simulink model "ap_12B"  (Simulink 8.0)
settings: Solver=ode3  StartTime=0.0  StopTime=100  FixedStep=Ts  RelTol=1e-3
undefined symbols (not defined in the file): beaver_b, beaver_c, beaver_mass, beaver_S, Cl0, Cl_alpha2_dpt, Cl_beta, Cl_da, Cl_da_alpha, Cl_dr, Cl_p, Cl_r, Cm0, Cm_alpha, Cm_alpha2, Cm_beta2, Cm_de, Cm_df, Cm_dpt, Cm_q, Cm_r, Cn0, Cn_beta, Cn_beta3, Cn_da, Cn_dpt3, Cn_dr, Cn_p, Cn_q, Cn_r, Cx0, Cx_alpha, Cx_alpha2, Cx_alpha3, Cx_df, Cx_df_alpha, Cx_dpt, Cx_dpt2_alpha, Cx_dr, Cx_q, Cy0, Cy_beta, Cy_da, Cy_dr, Cy_dr_alpha, Cy_p, Cy_r, Cz0, Cz_alpha, Cz_alpha3, Cz_de, Cz_de_beta, Cz_df, Cz_df_alpha, Cz_dpt, Cz_q, d2r, fin_act_1, fin_act_2, fin_act_3 ... (+23)
libraries: simulink x12, aerolibtransform2 x9, aerolibutil x7, aerolibasang x7, aerolibadynsys x3, aerolib6dofsys x2, aerolib6dof2 x1
(part 2 of 3)

== system ap_12B/DeHavilland Beaver Airframe/Aircraft Dynamics/Total Forces  and Moments ==
  EnvirBus : Inport
  Pilot : Inport  Port=2
  DCM : Inport  Port=3
  FltParams : Inport  Port=4
  Actuators : Subsystem
  Aerodynamics : Subsystem
  Bus Selector4 : BusSelector  OutputSignals=rho,g
  "Engine " : Subsystem
  Forces and Moments : Subsystem
  "Gravity " : Subsystem
  "Pilot " : InportShadow  Port=2
  Sum : Sum  Inputs=|++  SaturateOnIntegerOverflow=on  InputSameDT=on  OutDataTypeStr=Inherit: Same as first input
  Total Force : Outport
  Total Moment : Outport  Port=2
  wires:
  Forces and Moments/1(XYZ) -> Sum/1
  "Engine "/1(Engine Coefficients) -> Forces and Moments/3(Engine Coefficients)
  "Gravity "/1(Fgrav) -> Sum/2
  Aerodynamics/1(Aero Coefficients) -> Forces and Moments/1(Aero Coefficients)
  Pilot/1 -> Actuators/1(Pilot)
  Bus Selector4/1 -> "Engine "/3(rho)  "<rho>"
  DCM/1 -> "Gravity "/2(DCM)
  Bus Selector4/2 -> "Gravity "/1(g)  "<g>"
  Sum/1 -> Total Force/1  "Ftot"
  Forces and Moments/2(LMN) -> Total Moment/1  "Mtot"
  "Pilot "/1 -> "Engine "/2(Pilot)
  FltParams/1 -> Forces and Moments/2(Fltparams), "Engine "/1(Fltparams), Aerodynamics/2(FltParams)
  Actuators/1(uaero-out) -> Aerodynamics/1(Uaero)
  EnvirBus/1 -> Bus Selector4/1

== system ap_12B/DeHavilland Beaver Airframe/Calculate Parameters/ Incidence, Sideslip,  & Airspeed ==
  Vb : Inport
  Airspeed : Sqrt  AlgorithmType=Newton-Raphson  SaturateOnIntegerOverflow=on
  Incidence : Trigonometry  Operator=atan2
  Product : Product  Inputs=*/  SaturateOnIntegerOverflow=on  OutDataTypeStr=Inherit: Same as first input
  Sideslip : Trigonometry  Operator=asin
  Subsystem : aerolibasang/Incidence, Sideslip, & Airspeed/Subsystem
  Subsystem1 : aerolibasang/Incidence, Sideslip, & Airspeed/Subsystem1
  dot : aerolibasang/Incidence, Sideslip, & Airspeed/dot
  Alpha : Outport  InitialOutput=0
  Beta : Outport  Port=2  InitialOutput=0
  V : Outport  Port=3  InitialOutput=0
  wires:
  Sideslip/1 -> Beta/1
  Subsystem1/1 -> Product/1
  Product/1 -> Sideslip/1
  Subsystem/1 -> Incidence/1
  Subsystem/2 -> Incidence/2
  dot/1 -> Airspeed/1
  Airspeed/1 -> V/1, Product/2
  Incidence/1 -> Alpha/1
  Vb/1 -> Subsystem/1, dot/1, Subsystem1/1

== system ap_12B/DeHavilland Beaver Airframe/Calculate Parameters/Dynamic Pressure ==
  Velocity : Inport
  Air Density : Inport  Port=2
  1/2rhoV^2 : Gain  Gain=0.5  SaturateOnIntegerOverflow=on  OutDataTypeStr=Inherit: Same as input  ParamDataTypeStr=Inherit: Same as input
  Product2 : Product  SaturateOnIntegerOverflow=on  InputSameDT=on  OutDataTypeStr=Inherit: Same as first input
  dot : aerolibasang/Dynamic Pressure/dot
  qbar : Outport  InitialOutput=0
  wires:
  1/2rhoV^2/1 -> qbar/1
  Air Density/1 -> Product2/2
  dot/1 -> Product2/1
  Product2/1 -> 1/2rhoV^2/1
  Velocity/1 -> dot/1

== system ap_12B/Sensors/Air Data Sensor/ Incidence, Sideslip,  & Airspeed ==
  Vb : Inport
  Airspeed : Sqrt  AlgorithmType=Newton-Raphson  SaturateOnIntegerOverflow=on
  Gain : Gain  Gain=180/pi
  Gain1 : Gain  Gain=180/pi
  Incidence : Trigonometry  Operator=atan2
  Product : Product  Inputs=*/  SaturateOnIntegerOverflow=on  OutDataTypeStr=Inherit: Same as first input
  Scope : Scope
      settings: SaveName=ScopeData24
  Scope1 : Scope
      settings: SaveName=ScopeData25
  Sideslip : Trigonometry  Operator=asin
  Subsystem : aerolibasang/Incidence, Sideslip, & Airspeed/Subsystem
  Subsystem1 : aerolibasang/Incidence, Sideslip, & Airspeed/Subsystem1
  dot : aerolibasang/Incidence, Sideslip, & Airspeed/dot
  Alpha : Outport  InitialOutput=0
  Beta : Outport  Port=2  InitialOutput=0
  V : Outport  Port=3  InitialOutput=0
  wires:
  Sideslip/1 -> Gain1/1, Beta/1
  Subsystem1/1 -> Product/1
  Product/1 -> Sideslip/1
  Subsystem/1 -> Incidence/1
  Subsystem/2 -> Incidence/2
  dot/1 -> Airspeed/1
  Airspeed/1 -> V/1, Product/2
  Incidence/1 -> Gain/1, Alpha/1
  Vb/1 -> Subsystem/1, dot/1, Subsystem1/1
  Gain/1 -> Scope/1
  Gain1/1 -> Scope1/1

== system ap_12B/Sensors/Air Data Sensor/ic1 ==
  u : Inport
  ic : Inport  Port=2
  Constant : Constant
  Switch : Switch  Criteria=u2 ~= 0
  Unit Delay : UnitDelay  SampleTime=-1
  y : Outport
  wires:
  Switch/1 -> y/1
  u/1 -> Switch/1
  ic/1 -> Switch/3
  Constant/1 -> Unit Delay/1
  Unit Delay/1 -> Switch/2

== system ap_12B/Sensors/Air Data Sensor/ic2 ==
  u : Inport
  ic : Inport  Port=2
  Constant : Constant
  Switch : Switch  Criteria=u2 ~= 0
  Unit Delay : UnitDelay  SampleTime=-1
  y : Outport
  wires:
  ic/1 -> Switch/3
  u/1 -> Switch/1
  Switch/1 -> y/1
  Constant/1 -> Unit Delay/1
  Unit Delay/1 -> Switch/2

== system ap_12B/Sensors/Air Data Sensor/ic3 ==
  u : Inport
  ic : Inport  Port=2
  Constant1 : Constant
  Switch : Switch  Criteria=u2 ~= 0
  Unit Delay1 : UnitDelay  SampleTime=-1
  y : Outport
  wires:
  ic/1 -> Switch/3
  u/1 -> Switch/1
  Switch/1 -> y/1
  Constant1/1 -> Unit Delay1/1
  Unit Delay1/1 -> Switch/2

== system ap_12B/Sensors/Inertial Data Sensor/ic ==
  u : Inport
  ic : Inport  Port=2
  Constant : Constant
  Switch : Switch  Criteria=u2 ~= 0
  Unit Delay : UnitDelay  SampleTime=-1
  y : Outport
  wires:
  Switch/1 -> y/1
  u/1 -> Switch/1
  ic/1 -> Switch/3
  Constant/1 -> Unit Delay/1
  Unit Delay/1 -> Switch/2

== system ap_12B/Sensors/Inertial Data Sensor/ic1 ==
  u : Inport
  ic : Inport  Port=2
  Constant : Constant
  Switch : Switch  Criteria=u2 ~= 0
  Unit Delay : UnitDelay  SampleTime=-1
  y : Outport
  wires:
  ic/1 -> Switch/3
  u/1 -> Switch/1
  Switch/1 -> y/1
  Constant/1 -> Unit Delay/1
  Unit Delay/1 -> Switch/2

== system ap_12B/Sensors/Inertial Data Sensor/ic2 ==
  u : Inport
  ic : Inport  Port=2
  Constant : Constant
  Switch : Switch  Criteria=u2 ~= 0
  Unit Delay : UnitDelay  SampleTime=-1
  y : Outport
  wires:
  Switch/1 -> y/1
  u/1 -> Switch/1
  ic/1 -> Switch/3
  Constant/1 -> Unit Delay/1
  Unit Delay/1 -> Switch/2

== system ap_12B/Sensors/Inertial Data Sensor/ic3 ==
  u : Inport
  ic : Inport  Port=2
  Constant : Constant
  Switch : Switch  Criteria=u2 ~= 0
  Unit Delay : UnitDelay  SampleTime=-1
  y : Outport
  wires:
  ic/1 -> Switch/3
  u/1 -> Switch/1
  Switch/1 -> y/1
  Constant/1 -> Unit Delay/1
  Unit Delay/1 -> Switch/2

== system ap_12B/Autopilot/Pitch_Autopilot/Altitude Mode/Rate Limiter ==
  note: Y(k)
  note: U(k)
  up : Inport
  u : Inport  Port=2
  lo : Inport  Port=3
  Constant1 : Constant  Value=Ts
  Delay Input2 : UnitDelay  Description=Store in Global RAM  DisableCoverage=on  SampleTime=-1
  Difference Inputs1 : Sum  Description=Add in CPU  DisableCoverage=on  Inputs=+-  OutDataTypeStr=Inherit: Inherit via back propagation
  Difference Inputs2 : Sum  Description=Add in CPU  OutDataTypeStr=Inherit: Inherit via back propagation
  Saturation Dynamic : simulink/Discontinuities/Saturation Dynamic  OutMin=[]  OutMax=[]  OutDataTypeStr=Inherit: Same as second input  OutDataType=fixdt(1, 16)  OutScaling=2^-10  DoSatur=off
  delta fall limit : Product  DisableCoverage=on  Inputs=**  OutDataTypeStr=Inherit: Inherit via back propagation  SaturateOnIntegerOverflow=on
  delta rise limit : Product  DisableCoverage=on  Inputs=**  OutDataTypeStr=Inherit: Inherit via back propagation  SaturateOnIntegerOverflow=on
  Y : Outport  InitialOutput=0
  wires:
  Difference Inputs1/1 -> Saturation Dynamic/2  "( U(k) - Y(k-1) )"
  u/1 -> Difference Inputs1/1
  delta fall limit/1 -> Saturation Dynamic/3
  Saturation Dynamic/1 -> Difference Inputs2/1
  Delay Input2/1 -> Difference Inputs1/2, Difference Inputs2/2  "Y(k-1)"
  Difference Inputs2/1 -> Y/1, Delay Input2/1
  up/1 -> delta rise limit/1
  delta rise limit/1 -> Saturation Dynamic/1
  lo/1 -> delta fall limit/1
  Constant1/1 -> delta rise limit/2, delta fall limit/2

== system ap_12B/Autopilot/Pitch_Autopilot/Altitude Mode/ResetIntegratorInternal ==
  note: ic
  note: Level Reset Integration With Saturation
      | y(n) = y(n-1) + K*Ts*u(n-1)
  U : Inport
  R : Inport  Port=2
  IC : Inport  Port=3
  Constant : Constant  Value=0.2
  Constant1 : Constant  Value=Ts
  Product : Product  RndMeth=Zero
  Product1 : Product  RndMeth=Zero
  Saturation : Saturate  UpperLimit=20  LowerLimit=-20
  Sum3 : Sum
  Switch : Switch  Criteria=u2 ~= 0
  Switch1 : Switch  Criteria=u2 ~= 0
  X : UnitDelay  SampleTime=Ts
  Y : Outport
  wires:
  Product1/1 -> Sum3/1
  U/1 -> Product1/2
  Sum3/1 -> Switch1/3
  Product/1 -> Product1/1
  Switch/1 -> Saturation/1
  IC/1 -> Switch1/1, Switch/1
  Constant1/1 -> Product/2  "deltaT"
  Switch1/1 -> X/1
  Constant/1 -> Product/1  "gain"
  Saturation/1 -> Y/1, Sum3/2
  R/1 -> Switch1/2, Switch/2
  X/1 -> Switch/3

== system ap_12B/Autopilot/Pitch_Autopilot/Basic Pitch Mode/ResetIntegratorInternal ==
  note: ic
  note: Level Reset Integration With Saturation
      | y(n) = y(n-1) + K*Ts*u(n-1)
  U : Inport
  R : Inport  Port=2
  Constant : Constant  Value=1.0
  Constant1 : Constant  Value=Ts
  Constant2 : Constant  Value=0.0
  Product : Product  RndMeth=Zero
  Product1 : Product  RndMeth=Zero
  Saturation : Saturate  UpperLimit=5  LowerLimit=-5
  Sum3 : Sum
  Switch : Switch  Criteria=u2 ~= 0
  Switch1 : Switch  Criteria=u2 ~= 0
  X : UnitDelay  SampleTime=Ts
  Y : Outport
  wires:
  Product1/1 -> Sum3/1
  U/1 -> Product1/2
  Sum3/1 -> Switch1/3
  Product/1 -> Product1/1
  Switch/1 -> Saturation/1
  Constant2/1 -> Switch1/1, Switch/1
  Constant1/1 -> Product/2  "deltaT"
  Switch1/1 -> X/1
  Constant/1 -> Product/1  "gain"
  Saturation/1 -> Y/1, Sum3/2
  R/1 -> Switch1/2, Switch/2
  X/1 -> Switch/3

== system ap_12B/Autopilot/Pitch_Autopilot/Pitch Reference/latch ==
  note: Xold
  note: Enable
  u : Inport
  E : Inport  Port=2
  Enable : Switch  Criteria=u2 ~= 0  OutDataTypeStr=Inherit: Inherit via back propagation  ZeroCross=off
  FixPt Unit Delay1 : UnitDelay  SampleTime=Ts  HasFrameUpgradeWarning=off
  y : Outport
  wires:
  FixPt Unit Delay1/1 -> y/1, Enable/3
  Enable/1 -> FixPt Unit Delay1/1  "Xnew"
  E/1 -> Enable/2
  u/1 -> Enable/1

== system ap_12B/Autopilot/Roll_Autopilot/Basic Roll Mode/ResetIntegratorInternal ==
  note: ic
  note: Level Reset Integration With Saturation
      | y(n) = y(n-1) + K*Ts*u(n-1)
  U : Inport
  R : Inport  Port=2
  Constant : Constant  Value=1.0
  Constant1 : Constant  Value=Ts
  Constant2 : Constant  Value=0.0
  Product : Product  RndMeth=Zero
  Product1 : Product  RndMeth=Zero
  Saturation : Saturate  UpperLimit=5  LowerLimit=-5
  Sum3 : Sum
  Switch : Switch  Criteria=u2 ~= 0
  Switch1 : Switch  Criteria=u2 ~= 0
  X : UnitDelay  SampleTime=Ts
  Y : Outport
  wires:
  Product1/1 -> Sum3/1
  U/1 -> Product1/2
  Sum3/1 -> Switch1/3
  Product/1 -> Product1/1
  Switch/1 -> Saturation/1
  Constant2/1 -> Switch1/1, Switch/1
  Constant1/1 -> Product/2  "deltaT"
  Switch1/1 -> X/1
  Constant/1 -> Product/1  "gain"
  Saturation/1 -> Y/1, Sum3/2
  R/1 -> Switch1/2, Switch/2
  X/1 -> Switch/3

== system ap_12B/Autopilot/Roll_Autopilot/Heading Mode/angle diff ==
  plus : Inport  OutDataTypeStr=double
  minus : Inport  Port=2  OutDataTypeStr=double
  abs : Abs  ZeroCross=off
  constant : Constant  Value=180
  constant1 : Constant  Value=360
  floor : Rounding
  product : Product  RndMeth=Zero  InputSameDT=on  OutDataTypeStr=Inherit: Same as first input
  product1 : Product  Inputs=*/  RndMeth=Zero  InputSameDT=on  OutDataTypeStr=Inherit: Same as first input
  product2 : Product  RndMeth=Zero  InputSameDT=on  OutDataTypeStr=Inherit: Same as first input
  signum : Signum  ZeroCross=off
  sum : Sum  Inputs=|+-  RndMeth=Zero  InputSameDT=on  OutDataTypeStr=Inherit: Same as first input
  sum1 : Sum  Inputs=|+-  RndMeth=Zero  InputSameDT=on  OutDataTypeStr=Inherit: Same as first input
  sum2 : Sum  Inputs=|++  RndMeth=Zero  InputSameDT=on  OutDataTypeStr=Inherit: Same as first input
  diff : Outport
  wires:
  product2/1 -> product/2
  product/1 -> sum1/2
  sum2/1 -> product1/1
  constant/1 -> sum2/2
  sum1/1 -> diff/1
  signum/1 -> product/1
  floor/1 -> product2/1
  minus/1 -> sum/2
  plus/1 -> sum/1
  product1/1 -> floor/1
  sum/1 -> sum1/1, abs/1, signum/1
  abs/1 -> sum2/1
  constant1/1 -> product2/2, product1/2

== system ap_12B/Autopilot/Roll_Autopilot/Roll Reference/latch ==
  note: Xold
  note: Enable
  u : Inport
  E : Inport  Port=2
  Enable : Switch  Criteria=u2 ~= 0  OutDataTypeStr=Inherit: Inherit via back propagation  ZeroCross=off
  FixPt Unit Delay1 : UnitDelay  SampleTime=Ts  HasFrameUpgradeWarning=off
  y : Outport
  wires:
  FixPt Unit Delay1/1 -> y/1, Enable/3
  Enable/1 -> FixPt Unit Delay1/1  "Xnew"
  E/1 -> Enable/2
  u/1 -> Enable/1

== system ap_12B/DeHavilland Beaver Airframe/Aircraft Dynamics/6DoF (Quaternion)/3x3 CrossProduct ==
  A : Inport
  B : Inport  Port=2
  A_1 : InportShadow
  B_1 : InportShadow  Port=2
  Subsystem : aerolibutil/3x3 Cross Product/Subsystem
  Subsystem1 : aerolibutil/3x3 Cross Product/Subsystem1
  Sum : Sum  Inputs=+|-  SaturateOnIntegerOverflow=on  InputSameDT=on  OutDataTypeStr=Inherit: Same as first input
  C : Outport
  wires:
  Subsystem/1 -> Sum/1
  Subsystem1/1 -> Sum/2
  B/1 -> Subsystem/2
  A/1 -> Subsystem/1
  B_1/1 -> Subsystem1/2
  A_1/1 -> Subsystem1/1
  Sum/1 -> C/1

== system ap_12B/DeHavilland Beaver Airframe/Aircraft Dynamics/6DoF (Quaternion)/Calculate DCM & Euler Angles ==
  p q r : Inport
  Initial Euler Angles : Constant  Value="[0    0.1303    1.9722]"
  Quaternions to  Direction Cosine Matrix : Subsystem
  Quaternions to Rotation Angles (ZYX) : Subsystem
  ResetIntegratorInternal1 : Subsystem
  Rotation Angles to Quats (ZYX) : Subsystem
  Selector : Selector  InputPortWidth=3  IndexOptions=Index vector (dialog)  Indices=[3 2 1]  OutputSizes=1
  Selector1 : Selector  InputPortWidth=3  IndexOptions=Index vector (dialog)  Indices=[3 2 1]  OutputSizes=1
  ic3 : Subsystem
  qd : Subsystem
  DCM : Outport
  Euler : Outport  Port=2
  wires:
  Selector1/1 -> Rotation Angles to Quats (ZYX)/1("R1, R2, R3")
  Selector/1 -> Euler/1
  Quaternions to Rotation Angles (ZYX)/1(R1,R2,R3) -> Selector/1
  Quaternions to  Direction Cosine Matrix/1(DCM) -> DCM/1
  p q r/1 -> qd/1(p q r)
  Initial Euler Angles/1 -> Selector1/1
  ResetIntegratorInternal1/1(Y) -> Quaternions to  Direction Cosine Matrix/1(Quat), qd/2(q0 q1 q2 q3), Quaternions to Rotation Angles (ZYX)/1(q)
  qd/1(qdot) -> ResetIntegratorInternal1/1(U)
  ic3/1(R) -> ResetIntegratorInternal1/2(R)
  ic3/2(IC) -> ResetIntegratorInternal1/3(IC)
  Rotation Angles to Quats (ZYX)/1(Quat) -> ic3/1(ic)

== system ap_12B/DeHavilland Beaver Airframe/Aircraft Dynamics/6DoF (Quaternion)/Calculate omega_dot ==
  p q r : Inport
  "I, I_dot" : Inport  Port=2
  Moments : Inport  Port=3
  3x3 CrossProduct : Subsystem
  I x w : aerolib6dofsys/Calculate omega_dot/I x w
  I x w1 : aerolib6dofsys/Calculate omega_dot/I x w1
  Product2 : Product  Inputs=*/  Multiplication=Matrix(*)  SaturateOnIntegerOverflow=on  OutDataTypeStr=Inherit: Same as first input
  Reshape : Reshape
  Reshape1 : Reshape  OutputDimensionality=Row vector (2-D)
  Selector : Selector  NumberOfDimensions=2  InputPortWidth=2  IndexOptions=Index vector (dialog),Select all  Indices=1:3,-1  OutputSizes=1
  Selector1 : Selector  NumberOfDimensions=2  InputPortWidth=2  IndexOptions=Index vector (dialog),Select all  Indices=4:6,-1  OutputSizes=1
  Selector2 : Selector  NumberOfDimensions=2  InputPortWidth=2  IndexOptions=Index vector (dialog),Select all  Indices=1:3,-1  OutputSizes=1
  Sum2 : Sum  Inputs=+--  SaturateOnIntegerOverflow=on
  pdot qdot rdot : Outport
  wires:
  Reshape1/1 -> Product2/1
  I x w/1 -> 3x3 CrossProduct/2(B)
  3x3 CrossProduct/1(C) -> Sum2/3
  Selector1/1 -> I x w1/1
  I x w1/1 -> Sum2/2
  Moments/1 -> Sum2/1
  Sum2/1 -> Reshape1/1
  Product2/1 -> Reshape/1
  p q r/1 -> 3x3 CrossProduct/1(A), I x w1/2, I x w/1
  "I, I_dot"/1 -> Selector2/1, Selector/1, Selector1/1
  Selector2/1 -> Product2/2
  Selector/1 -> I x w/2
  Reshape/1 -> pdot qdot rdot/1

== system ap_12B/DeHavilland Beaver Airframe/Aircraft Dynamics/6DoF (Quaternion)/ResetIntegratorInternal ==
  note: ic
  note: Level Reset Integration With Saturation
      | y(n) = y(n-1) + K*Ts*u(n-1)
  U : Inport
  R : Inport  Port=2
  IC : Inport  Port=3
  Constant : Constant  Value=1.0
  Constant1 : Constant  Value=Ts
  Product : Product  RndMeth=Zero
  Product1 : Product  RndMeth=Zero
  Sum3 : Sum
  Switch : Switch  Criteria=u2 ~= 0
  Switch1 : Switch  Criteria=u2 ~= 0
  X : UnitDelay  SampleTime=Ts
  Y : Outport
  wires:
  Product1/1 -> Sum3/1
  U/1 -> Product1/2
  Sum3/1 -> Switch1/3
  Product/1 -> Product1/1
  IC/1 -> Switch1/1, Switch/1
  Constant1/1 -> Product/2  "deltaT"
  Switch1/1 -> X/1
  Constant/1 -> Product/1  "gain"
  Switch/1 -> Y/1, Sum3/2
  R/1 -> Switch1/2, Switch/2
  X/1 -> Switch/3

== system ap_12B/DeHavilland Beaver Airframe/Aircraft Dynamics/6DoF (Quaternion)/ResetIntegratorInternal1 ==
  note: ic
  note: Level Reset Integration With Saturation
      | y(n) = y(n-1) + K*Ts*u(n-1)
  U : Inport
  R : Inport  Port=2
  IC : Inport  Port=3
  Constant : Constant  Value=1.0
  Constant1 : Constant  Value=Ts
  Product : Product  RndMeth=Zero
  Product1 : Product  RndMeth=Zero
  Sum3 : Sum
  Switch : Switch  Criteria=u2 ~= 0
  Switch1 : Switch  Criteria=u2 ~= 0
  X : UnitDelay  SampleTime=Ts
  Y : Outport
  wires:
  Product1/1 -> Sum3/1
  U/1 -> Product1/2
  Sum3/1 -> Switch1/3
  Product/1 -> Product1/1
  IC/1 -> Switch1/1, Switch/1
  Constant1/1 -> Product/2  "deltaT"
  Switch1/1 -> X/1
  Constant/1 -> Product/1  "gain"
  Switch/1 -> Y/1, Sum3/2
  R/1 -> Switch1/2, Switch/2
  X/1 -> Switch/3

== system ap_12B/DeHavilland Beaver Airframe/Aircraft Dynamics/6DoF (Quaternion)/ResetIntegratorInternal2 ==
  note: Level Reset Integration With Saturation
      | y(n) = y(n-1) + K*Ts*u(n-1)
  note: ic
  U : Inport
  R : Inport  Port=2
  IC : Inport  Port=3
  Constant : Constant  Value=1.0
  Constant1 : Constant  Value=Ts
  Product : Product  RndMeth=Zero
  Product1 : Product  RndMeth=Zero
  Sum3 : Sum
  Switch : Switch  Criteria=u2 ~= 0
  Switch1 : Switch  Criteria=u2 ~= 0
  X : UnitDelay  SampleTime=Ts
  Y : Outport
  wires:
  X/1 -> Switch/3
  R/1 -> Switch/2, Switch1/2
  Constant/1 -> Product/1  "gain"
  Switch1/1 -> X/1
  Constant1/1 -> Product/2  "deltaT"
  IC/1 -> Switch/1, Switch1/1
  Product/1 -> Product1/1
  Sum3/1 -> Switch1/3
  U/1 -> Product1/2
  Product1/1 -> Sum3/1
  Switch/1 -> Sum3/2, Y/1

== system ap_12B/DeHavilland Beaver Airframe/Aircraft Dynamics/6DoF (Quaternion)/Subsystem ==
  Vb : Inport
  forces : Inport  Port=2
  "mass " : Inport  Port=3
  m_dot : Inport  Port=4  OutDataTypeStr=double
  I : Inport  Port=5  OutDataTypeStr=double
  I_dot : Inport  Port=6  OutDataTypeStr=double
  Constant : Constant  Value=beaver_mass  OutDataTypeStr=Inherit: Inherit via back propagation
  Constant1 : Constant  Value=[inertia; zeros(3,3)]  OutDataTypeStr=Inherit: Inherit via back propagation
  Ground : Ground
  Terminator{,1..4} (5 alike) : Terminator
  "forces " : Outport
  mass : Outport  Port=2
  "inertia, 0" : Outport  Port=3
  Out9 : Outport  Port=4
  wires:
  Constant1/1 -> "inertia, 0"/1
  "mass "/1 -> Terminator3/1
  forces/1 -> "forces "/1
  Vb/1 -> Terminator4/1
  Constant/1 -> mass/1
  I_dot/1 -> Terminator2/1
  I/1 -> Terminator/1
  Ground/1 -> Out9/1
  m_dot/1 -> Terminator1/1

== system ap_12B/DeHavilland Beaver Airframe/Aircraft Dynamics/6DoF (Quaternion)/ic1 ==
  Constant : Constant  Value=0
  Constant1 : Constant  Value=xme_0
  Unit Delay : UnitDelay  InitialCondition=1  SampleTime=-1
  R : Outport
  IC : Outport  Port=2
  wires:
  Constant/1 -> Unit Delay/1
  Unit Delay/1 -> R/1
  Constant1/1 -> IC/1

== system ap_12B/DeHavilland Beaver Airframe/Aircraft Dynamics/6DoF (Quaternion)/ic2 ==
  Constant : Constant  Value=0
  Constant1 : Constant  Value=[44.54;2.714;5.836]
  Unit Delay : UnitDelay  InitialCondition=1  SampleTime=-1
  R : Outport
  IC : Outport  Port=2
  wires:
  Constant1/1 -> IC/1
  Constant/1 -> Unit Delay/1
  Unit Delay/1 -> R/1

== system ap_12B/DeHavilland Beaver Airframe/Aircraft Dynamics/6DoF (Quaternion)/ic3 ==
  Constant : Constant  Value=0
  Constant1 : Constant  Value=0
  Unit Delay : UnitDelay  InitialCondition=1  SampleTime=-1
  R : Outport
  IC : Outport  Port=2
  wires:
  Constant/1 -> Unit Delay/1
  Unit Delay/1 -> R/1
  Constant1/1 -> IC/1

== system ap_12B/DeHavilland Beaver Airframe/Aircraft Dynamics/Total Forces  and Moments/Actuators ==
  Pilot : Inport
  Bus Selector2 : BusSelector  OutputSignals=uaero
  Demux : Demux
  Initial inputs for aero : Constant  Value=uaero0
  Mux : Mux
  Scope : Scope
      settings: SaveName=ScopeData13
  Sum1 : Sum  Inputs=++|  SaturateOnIntegerOverflow=on  InputSameDT=on  OutDataTypeStr=Inherit: Same as first input
  sof : Subsystem
  sof1 : Subsystem
  sof2 : Subsystem
  uaero-out : Outport
  wires:
  Pilot/1 -> Bus Selector2/1
  Initial inputs for aero/1 -> Sum1/1
  Demux/4 -> Mux/4
  Demux/1 -> sof/1(Ac_dem)
  Demux/2 -> sof1/1(Ac_dem)
  Sum1/1 -> Demux/1
  sof/1(Ac_ac) -> Mux/1
  sof1/1(Ac_ac) -> Mux/2
  Bus Selector2/1 -> Sum1/2  "<uaero>"
  Mux/1 -> Scope/1, uaero-out/1
  Demux/3 -> sof2/1(Ac_dem)
  sof2/1(Ac_ac) -> Mux/3

== system ap_12B/DeHavilland Beaver Airframe/Aircraft Dynamics/Total Forces  and Moments/Aerodynamics ==
  Uaero : Inport
  FltParams : Inport  Port=2
  Actuator Increments : Subsystem
  Body Rate Damping : Subsystem
  Bus Selector1 : BusSelector  OutputSignals=alpha,beta
  Bus Selector2 : BusSelector  OutputSignals=V,pqr_tot
  Datum Coefficients : Subsystem
  Sum1 : Sum  Inputs=|++  SaturateOnIntegerOverflow=on
  Sum4 : Sum  Inputs=|++  SaturateOnIntegerOverflow=on
  Aero Coefficients : Outport
  wires:
  Bus Selector1/2 -> Actuator Increments/2(beta), Datum Coefficients/2(beta)  "<beta>"
  Bus Selector2/1 -> Body Rate Damping/1(V)  "<V>"
  Bus Selector2/2 -> Body Rate Damping/2(p,q,r)  "<pqr_tot>"
  Uaero/1 -> Actuator Increments/3(Actuator Deflections)
  Bus Selector1/1 -> Actuator Increments/1(alpha), Datum Coefficients/1(alpha)  "<alpha>"
  FltParams/1 -> Bus Selector1/1, Bus Selector2/1
  Datum Coefficients/1(Coefficients) -> Sum4/1
  Actuator Increments/1(Coefficients) -> Sum4/2
  Sum4/1 -> Sum1/1
  Body Rate Damping/1(Coefficients) -> Sum1/2
  Sum1/1 -> Aero Coefficients/1

== system ap_12B/DeHavilland Beaver Airframe/Aircraft Dynamics/Total Forces  and Moments/Engine  ==
  Fltparams : Inport
  Pilot : Inport  Port=2
  rho : Inport  Port=3
  Bus Selector4 : BusSelector  OutputSignals=V,alpha
  eng : Subsystem
  pow : Subsystem
  Engine Coefficients : Outport
  wires:
  Bus Selector4/1 -> pow/3(V)  "<V>"
  rho/1 -> pow/1(rho)
  Bus Selector4/2 -> eng/2(alpha)  "<alpha>"
  eng/1(Cprop) -> Engine Coefficients/1
  Pilot/1 -> pow/2(Pilot)
  pow/1(dpt) -> eng/1(dpt)
  Fltparams/1 -> Bus Selector4/1

== system ap_12B/DeHavilland Beaver Airframe/Aircraft Dynamics/Total Forces  and Moments/Forces and Moments ==
  Aero Coefficients : Inport
  Fltparams : Inport  Port=2
  Engine Coefficients : Inport  Port=3
  Aero F&M : Subsystem
  Bus Selector4 : BusSelector  OutputSignals=Qdyn
  Scope : Scope
      settings: SaveName=ScopeData22
  Sum : Sum  Inputs=++|  SaturateOnIntegerOverflow=on  InputSameDT=on  OutDataTypeStr=Inherit: Same as first input
  neglect center of gravity  and center of pressure effects : Constant  Value=[0 0 0]
  XYZ : Outport
  LMN : Outport  Port=2
  wires:
  Sum/1 -> Aero F&M/1(Coefficients)
  Aero Coefficients/1 -> Sum/2
  Engine Coefficients/1 -> Sum/1
  Fltparams/1 -> Bus Selector4/1
  Aero F&M/1(Forces) -> XYZ/1
  neglect center of gravity  and center of pressure effects/1 -> Aero F&M/4(CP), Aero F&M/3(CG)
  Bus Selector4/1 -> Scope/1, Aero F&M/2(qbar)  "<Qdyn>"
  Aero F&M/2(Moments) -> LMN/1

== system ap_12B/DeHavilland Beaver Airframe/Aircraft Dynamics/Total Forces  and Moments/Gravity  ==
  g : Inport
  DCM : Inport  Port=2
  Constant : Constant  Value=0.0
  Gain : Gain  Gain=beaver_mass
  Inertial to Body : Product  Multiplication=Matrix(*)  SaturateOnIntegerOverflow=on  InputSameDT=on  OutDataTypeStr=Inherit: Same as first input
  Mux : Mux  Inputs=3
  Reshape1 : Reshape
  Fgrav : Outport
  wires:
  Inertial to Body/1 -> Reshape1/1
  g/1 -> Gain/1
  DCM/1 -> Inertial to Body/1
  Mux/1 -> Inertial to Body/2
  Reshape1/1 -> Fgrav/1
  Constant/1 -> Mux/2, Mux/1
  Gain/1 -> Mux/3

== system ap_12B/DeHavilland Beaver Airframe/Aircraft Dynamics/6DoF (Quaternion)/Calculate DCM & Euler Angles/Quaternions to  Direction Cosine Matrix ==
  Quat : Inport  PortDimensions=4
  A11 : aerolibtransform2/Quaternions to  Direction Cosine Matrix/A11
  A12 : aerolibtransform2/Quaternions to  Direction Cosine Matrix/A12
  A13 : aerolibtransform2/Quaternions to  Direction Cosine Matrix/A13
  A21 : aerolibtransform2/Quaternions to  Direction Cosine Matrix/A21
  A22 : aerolibtransform2/Quaternions to  Direction Cosine Matrix/A22
  A23 : aerolibtransform2/Quaternions to  Direction Cosine Matrix/A23
  A31 : aerolibtransform2/Quaternions to  Direction Cosine Matrix/A31
  A32 : aerolibtransform2/Quaternions to  Direction Cosine Matrix/A32
  A33 : aerolibtransform2/Quaternions to  Direction Cosine Matrix/A33
  Create Transformation Matrix : aerolibutil/Create 3x3 Matrix
  Quaternion Normalize : Subsystem
  DCM : Outport  PortDimensions=[3,3]  InitialOutput=0
  wires:
  Create Transformation Matrix/1 -> DCM/1
  A11/1 -> Create Transformation Matrix/1
  A21/1 -> Create Transformation Matrix/4
  A31/1 -> Create Transformation Matrix/7
  A32/1 -> Create Transformation Matrix/8
  A13/1 -> Create Transformation Matrix/3
  A23/1 -> Create Transformation Matrix/6
  A33/1 -> Create Transformation Matrix/9
  Quat/1 -> Quaternion Normalize/1(q)
  Quaternion Normalize/1(normal(q)) -> A33/1, A32/1, A31/1, A23/1, A22/1, A21/1, A13/1, A12/1, A11/1
  A22/1 -> Create Transformation Matrix/5
  A12/1 -> Create Transformation Matrix/2

== system ap_12B/DeHavilland Beaver Airframe/Aircraft Dynamics/6DoF (Quaternion)/Calculate DCM & Euler Angles/Quaternions to Rotation Angles (ZYX) ==
  q : Inport
  Quaternion Normalize : Subsystem
  Trigonometric Function1 : Trigonometry  Operator=atan2
  Trigonometric Function3 : Trigonometry  Operator=atan2
  Vector Concatenate : Concatenate  NumInputs=3
  fcn1 : Fcn  Expr=2*(u[2]*u[3] + u[1]*u[4])
  fcn2 : Fcn  Expr=u[1]*u[1] + u[2]*u[2] - u[3]*u[3] - u[4]*u[4]
  fcn3 : Fcn  Expr=-2*(u[2]*u[4] - u[1]*u[3])
  fcn4 : Fcn  Expr=2*(u[3]*u[4] + u[1]*u[2])
  fcn5 : Fcn  Expr=u[1]*u[1] - u[2]*u[2] - u[3]*u[3] + u[4]*u[4]
  trigFcn : Trigonometry  Operator=asin
  R1,R2,R3 : Outport
  wires:
  fcn5/1 -> Trigonometric Function3/2
  fcn4/1 -> Trigonometric Function3/1
  fcn2/1 -> Trigonometric Function1/2
  fcn3/1 -> trigFcn/1
  q/1 -> Quaternion Normalize/1(q)
  Vector Concatenate/1 -> R1,R2,R3/1
  Trigonometric Function3/1 -> Vector Concatenate/3  "r3"
  Trigonometric Function1/1 -> Vector Concatenate/1  "r1"
  Quaternion Normalize/1(normal(q)) -> fcn1/1, fcn2/1, fcn5/1, fcn4/1, fcn3/1
  trigFcn/1 -> Vector Concatenate/2  "r2"
  fcn1/1 -> Trigonometric Function1/1

== system ap_12B/DeHavilland Beaver Airframe/Aircraft Dynamics/6DoF (Quaternion)/Calculate DCM & Euler Angles/ResetIntegratorInternal1 ==
  note: ic
  note: Level Reset Integration With Saturation
      | y(n) = y(n-1) + K*Ts*u(n-1)
  U : Inport
  R : Inport  Port=2
  IC : Inport  Port=3
  Constant : Constant  Value=1.0
  Constant1 : Constant  Value=Ts
  Product : Product  RndMeth=Zero
  Product1 : Product  RndMeth=Zero
  Saturation : Saturate  UpperLimit=20  LowerLimit=-20
  Sum3 : Sum
  Switch : Switch  Criteria=u2 ~= 0
  Switch1 : Switch  Criteria=u2 ~= 0
  X : UnitDelay  SampleTime=Ts
  Y : Outport
  wires:
  Product1/1 -> Sum3/1
  U/1 -> Product1/2
  Sum3/1 -> Switch1/3
  Product/1 -> Product1/1
  Switch/1 -> Saturation/1
  IC/1 -> Switch1/1, Switch/1
  Constant1/1 -> Product/2  "deltaT"
  Switch1/1 -> X/1
  Constant/1 -> Product/1  "gain"
  Saturation/1 -> Y/1, Sum3/2
  R/1 -> Switch1/2, Switch/2
  X/1 -> Switch/3

== system ap_12B/DeHavilland Beaver Airframe/Aircraft Dynamics/6DoF (Quaternion)/Calculate DCM & Euler Angles/Rotation Angles to Quats (ZYX) ==
  "R1, R2, R3" : Inport
  1/2 : Gain  Gain=0.5  SaturateOnIntegerOverflow=on  OutDataTypeStr=Inherit: Same as input  ParamDataTypeStr=Inherit: Same as input
  Mux1 : Mux  Inputs=2
  Mux2 : Mux
  q0 : Fcn  Expr=u(4)*u(5)*u(6) + u(1)*u(2)*u(3)
  q1 : Fcn  Expr=u(4)*u(5)*u(3) - u(1)*u(2)*u(6)
  q2 : Fcn  Expr=u(4)*u(2)*u(6) + u(1)*u(5)*u(3)
  q3 : Fcn  Expr=u(1)*u(5)*u(6) - u(4)*u(2)*u(3)
  sincos : Trigonometry  Operator=sincos
  Quat : Outport  InitialOutput=0
  wires:
  sincos/1 -> Mux1/1
  1/2/1 -> sincos/1
  "R1, R2, R3"/1 -> 1/2/1
  sincos/2 -> Mux1/2
  Mux1/1 -> q0/1, q1/1, q2/1, q3/1
  q1/1 -> Mux2/2
  q2/1 -> Mux2/3
  q3/1 -> Mux2/4
  Mux2/1 -> Quat/1
  q0/1 -> Mux2/1

== system ap_12B/DeHavilland Beaver Airframe/Aircraft Dynamics/6DoF (Quaternion)/Calculate DCM & Euler Angles/ic3 ==
  ic : Inport
  Constant : Constant  Value=0
  Unit Delay : UnitDelay  InitialCondition=1  SampleTime=-1
  R : Outport
  IC : Outport  Port=2
  wires:
  Constant/1 -> Unit Delay/1
  Unit Delay/1 -> R/1
  ic/1 -> IC/1

== system ap_12B/DeHavilland Beaver Airframe/Aircraft Dynamics/6DoF (Quaternion)/Calculate DCM & Euler Angles/qd ==
  p q r : Inport
  q0 q1 q2 q3 : Inport  Port=2
  Constant : Constant
  Dot Product : DotProduct  OutDataTypeStr=Inherit: Inherit via internal rule
  High Gain Quaternion Normalization : Gain  Gain=1.0  SaturateOnIntegerOverflow=on  OutDataTypeStr=Inherit: Same as input  ParamDataTypeStr=Inherit: Same as input
  Mux1 : Mux  Inputs=[3 4 1]
  Mux2 : Mux
  Sum : Sum  Inputs=|+-  SaturateOnIntegerOverflow=on  InputSameDT=on  OutDataTypeStr=Inherit: Same as first input
  q0dot : Fcn  Expr=-0.5 * ( u[5]*u[1]+u[6]*u[2]+u[7]*u[3] ) + u[8]*u[4]
  q1dot : Fcn  Expr=0.5 * ( u[4]*u[1]+u[6]*u[3]-u[7]*u[2] ) + u[8]*u[5]
  q2dot : Fcn  Expr=0.5 * ( u[4]*u[2]+u[7]*u[1]-u[5]*u[3] ) + u[8]*u[6]
  q3dot : Fcn  Expr=0.5 * ( u[4]*u[3]+u[5]*u[2]-u[6]*u[1] ) + u[8]*u[7]
  qdot : Outport  InitialOutput=0
  wires:
  p q r/1 -> Mux1/1
  q3dot/1 -> Mux2/4
  q2dot/1 -> Mux2/3
  q1dot/1 -> Mux2/2
  Constant/1 -> Sum/1
  Mux1/1 -> q2dot/1, q3dot/1, q0dot/1, q1dot/1
  q0dot/1 -> Mux2/1
  Mux2/1 -> qdot/1
  Sum/1 -> High Gain Quaternion Normalization/1
  Dot Product/1 -> Sum/2
  High Gain Quaternion Normalization/1 -> Mux1/3
  q0 q1 q2 q3/1 -> Dot Product/1, Dot Product/2, Mux1/2

== system ap_12B/DeHavilland Beaver Airframe/Aircraft Dynamics/6DoF (Quaternion)/Calculate omega_dot/3x3 CrossProduct ==
  A : Inport
  B : Inport  Port=2
  A_1 : InportShadow
  B_1 : InportShadow  Port=2
  Subsystem : aerolibutil/3x3 Cross Product/Subsystem
  Subsystem1 : aerolibutil/3x3 Cross Product/Subsystem1
  Sum : Sum  Inputs=+|-  SaturateOnIntegerOverflow=on  InputSameDT=on  OutDataTypeStr=Inherit: Same as first input
  C : Outport
  wires:
  Subsystem/1 -> Sum/1
  Subsystem1/1 -> Sum/2
  B/1 -> Subsystem/2
  A/1 -> Subsystem/1
  B_1/1 -> Subsystem1/2
  A_1/1 -> Subsystem1/1
  Sum/1 -> C/1

== system ap_12B/DeHavilland Beaver Airframe/Aircraft Dynamics/Total Forces  and Moments/Actuators/sof ==
  Ac_dem : Inport
  2*zeta * wn : Gain  Gain=2.0 * z_fin* wn_fin  SaturateOnIntegerOverflow=on  OutDataTypeStr=Inherit: Same as input  ParamDataTypeStr=Inherit: Same as input
  Demand limits : Saturate  UpperLimit=fin_max  LowerLimit=fin_min
  ResetIntegratorInternal : Subsystem
  ResetIntegratorInternal1 : Subsystem
  Sum2 : Sum  Inputs=|+-  SaturateOnIntegerOverflow=on  InputSameDT=on  OutDataTypeStr=Inherit: Same as first input
  Sum3 : Sum  Inputs=|+-  SaturateOnIntegerOverflow=on  InputSameDT=on  OutDataTypeStr=Inherit: Same as first input
  ic1 : Subsystem
  ic3 : Subsystem
  rate limit*2*zeta/wn : Saturate  UpperLimit=fin_maxrate*2*z_fin/wn_fin  LowerLimit=-fin_maxrate*2*z_fin/wn_fin
  wn^2 : Gain  Gain=wn_fin* wn_fin  SaturateOnIntegerOverflow=on  OutDataTypeStr=Inherit: Same as input  ParamDataTypeStr=Inherit: Same as input
  Ac_ac : Outport  InitialOutput=0
  wires:
  ResetIntegratorInternal1/1(Y) -> Ac_ac/1, Sum3/2
  wn^2/1 -> Sum2/1
  ResetIntegratorInternal/1(Y) -> ResetIntegratorInternal1/1(U), 2*zeta * wn/1
  Sum2/1 -> ResetIntegratorInternal/1(U)
  Demand limits/1 -> Sum3/1
  rate limit*2*zeta/wn/1 -> wn^2/1
  Ac_dem/1 -> Demand limits/1
  Sum3/1 -> rate limit*2*zeta/wn/1
  2*zeta * wn/1 -> Sum2/2
  ic3/2(IC) -> ResetIntegratorInternal/3(ic)
  ic3/1(R) -> ResetIntegratorInternal/2(R)
  ic1/1(R) -> ResetIntegratorInternal1/2(R)
  ic1/2(IC) -> ResetIntegratorInternal1/3(ic)

== system ap_12B/DeHavilland Beaver Airframe/Aircraft Dynamics/Total Forces  and Moments/Actuators/sof1 ==
  Ac_dem : Inport
  2*zeta * wn : Gain  Gain=2.0 * z_fin* wn_fin  SaturateOnIntegerOverflow=on  OutDataTypeStr=Inherit: Same as input  ParamDataTypeStr=Inherit: Same as input
  Demand limits : Saturate  UpperLimit=fin_max  LowerLimit=fin_min
  ResetIntegratorInternal : Subsystem
  ResetIntegratorInternal1 : Subsystem
  Sum2 : Sum  Inputs=|+-  SaturateOnIntegerOverflow=on  InputSameDT=on  OutDataTypeStr=Inherit: Same as first input
  Sum3 : Sum  Inputs=|+-  SaturateOnIntegerOverflow=on  InputSameDT=on  OutDataTypeStr=Inherit: Same as first input
  ic1 : Subsystem
  ic3 : Subsystem
  rate limit*2*zeta/wn : Saturate  UpperLimit=fin_maxrate*2*z_fin/wn_fin  LowerLimit=-fin_maxrate*2*z_fin/wn_fin
  wn^2 : Gain  Gain=wn_fin* wn_fin  SaturateOnIntegerOverflow=on  OutDataTypeStr=Inherit: Same as input  ParamDataTypeStr=Inherit: Same as input
  Ac_ac : Outport  InitialOutput=0
  wires:
  ic1/2(IC) -> ResetIntegratorInternal1/3(ic)
  ic1/1(R) -> ResetIntegratorInternal1/2(R)
  ic3/1(R) -> ResetIntegratorInternal/2(R)
  ic3/2(IC) -> ResetIntegratorInternal/3(ic)
  2*zeta * wn/1 -> Sum2/2
  Sum3/1 -> rate limit*2*zeta/wn/1
  Ac_dem/1 -> Demand limits/1
  rate limit*2*zeta/wn/1 -> wn^2/1
  Demand limits/1 -> Sum3/1
  Sum2/1 -> ResetIntegratorInternal/1(U)
  ResetIntegratorInternal/1(Y) -> 2*zeta * wn/1, ResetIntegratorInternal1/1(U)
  wn^2/1 -> Sum2/1
  ResetIntegratorInternal1/1(Y) -> Sum3/2, Ac_ac/1

== system ap_12B/DeHavilland Beaver Airframe/Aircraft Dynamics/Total Forces  and Moments/Actuators/sof2 ==
  Ac_dem : Inport
  2*zeta * wn : Gain  Gain=2.0 * z_fin* wn_fin  SaturateOnIntegerOverflow=on  OutDataTypeStr=Inherit: Same as input  ParamDataTypeStr=Inherit: Same as input
  Demand limits : Saturate  UpperLimit=fin_max  LowerLimit=fin_min
  ResetIntegratorInternal : Subsystem
  ResetIntegratorInternal1 : Subsystem
  Sum2 : Sum  Inputs=|+-  SaturateOnIntegerOverflow=on  InputSameDT=on  OutDataTypeStr=Inherit: Same as first input
  Sum3 : Sum  Inputs=|+-  SaturateOnIntegerOverflow=on  InputSameDT=on  OutDataTypeStr=Inherit: Same as first input
  ic1 : Subsystem
  ic3 : Subsystem
  rate limit*2*zeta/wn : Saturate  UpperLimit=fin_maxrate*2*z_fin/wn_fin  LowerLimit=-fin_maxrate*2*z_fin/wn_fin
  wn^2 : Gain  Gain=wn_fin* wn_fin  SaturateOnIntegerOverflow=on  OutDataTypeStr=Inherit: Same as input  ParamDataTypeStr=Inherit: Same as input
  Ac_ac : Outport  InitialOutput=0
  wires:
  ResetIntegratorInternal1/1(Y) -> Ac_ac/1, Sum3/2
  wn^2/1 -> Sum2/1
  ResetIntegratorInternal/1(Y) -> ResetIntegratorInternal1/1(U), 2*zeta * wn/1
  Sum2/1 -> ResetIntegratorInternal/1(U)
  Demand limits/1 -> Sum3/1
  rate limit*2*zeta/wn/1 -> wn^2/1
  Ac_dem/1 -> Demand limits/1
  Sum3/1 -> rate limit*2*zeta/wn/1
  2*zeta * wn/1 -> Sum2/2
  ic3/2(IC) -> ResetIntegratorInternal/3(ic)
  ic3/1(R) -> ResetIntegratorInternal/2(R)
  ic1/1(R) -> ResetIntegratorInternal1/2(R)
  ic1/2(IC) -> ResetIntegratorInternal1/3(ic)

== system ap_12B/DeHavilland Beaver Airframe/Aircraft Dynamics/Total Forces  and Moments/Aerodynamics/Actuator Increments ==
  alpha : Inport
  beta : Inport  Port=2
  Actuator Deflections : Inport  Port=3
  Aileron : Subsystem
  Elevator : Subsystem
  Flap : Subsystem
  Rudder : Subsystem
  Sum1 : Sum  SaturateOnIntegerOverflow=on
  Sum2 : Sum  SaturateOnIntegerOverflow=on
  Sum3 : Sum  SaturateOnIntegerOverflow=on
  Coefficients : Outport
  wires:
  Actuator Deflections/1 -> Flap/2(Actuators), Aileron/2(Actuators), Elevator/1(Actuators), Rudder/2(Actuators)
  alpha/1 -> Flap/1(Alpha), Rudder/1(Alpha), Aileron/1(alpha)
  beta/1 -> Elevator/2(Beta)
  Aileron/1(delCoeff) -> Sum1/1
  Elevator/1(delCoeff) -> Sum1/2
  Rudder/1(delCoeff) -> Sum2/2
  Flap/1(delCoeff) -> Sum3/2
  Sum3/1 -> Coefficients/1
  Sum1/1 -> Sum2/1
  Sum2/1 -> Sum3/1

== system ap_12B/DeHavilland Beaver Airframe/Aircraft Dynamics/Total Forces  and Moments/Aerodynamics/Body Rate Damping ==
  V : Inport
  p,q,r : Inport  Port=2
  Demux : Demux  Outputs=3
  Product : Product  SaturateOnIntegerOverflow=on  InputSameDT=on  OutDataTypeStr=Inherit: Same as first input
  Product1 : Product  SaturateOnIntegerOverflow=on  InputSameDT=on  OutDataTypeStr=Inherit: Same as first input
  Product2 : Product  SaturateOnIntegerOverflow=on  InputSameDT=on  OutDataTypeStr=Inherit: Same as first input
  Product3 : Product  Inputs=*/  SaturateOnIntegerOverflow=on  InputSameDT=on  OutDataTypeStr=Inherit: Same as first input
  Reference Length : Gain  Gain=beaver_c  SaturateOnIntegerOverflow=on  OutDataTypeStr=Inherit: Same as input  ParamDataTypeStr=Inherit: Same as input
  Reference Span : Gain  Gain=beaver_b/2  SaturateOnIntegerOverflow=on  OutDataTypeStr=Inherit: Same as input  ParamDataTypeStr=Inherit: Same as input
  "Reference Span " : Gain  Gain=beaver_b/2  SaturateOnIntegerOverflow=on  OutDataTypeStr=Inherit: Same as input  ParamDataTypeStr=Inherit: Same as input
  Sum1 : Sum  SaturateOnIntegerOverflow=on
  Sum2 : Sum  SaturateOnIntegerOverflow=on
  p : Subsystem
  q : Subsystem
  r : Subsystem
  Coefficients : Outport
  wires:
  p/1(delCoeff) -> Product/1
  q/1(delCoeff) -> Product1/1
  p,q,r/1 -> Demux/1
  Demux/1 -> Product/2  "p"
  Demux/2 -> Product1/2  "q"
  Demux/3 -> Product2/2  "r"
  Sum1/1 -> Product3/1
  V/1 -> Product3/2
  Product3/1 -> Coefficients/1
  Product1/1 -> Reference Length/1
  Product2/1 -> "Reference Span "/1
  Product/1 -> Reference Span/1
  r/1(delCoeff) -> Product2/1
  Reference Length/1 -> Sum2/2
  "Reference Span "/1 -> Sum1/2
  Reference Span/1 -> Sum2/1
  Sum2/1 -> Sum1/1

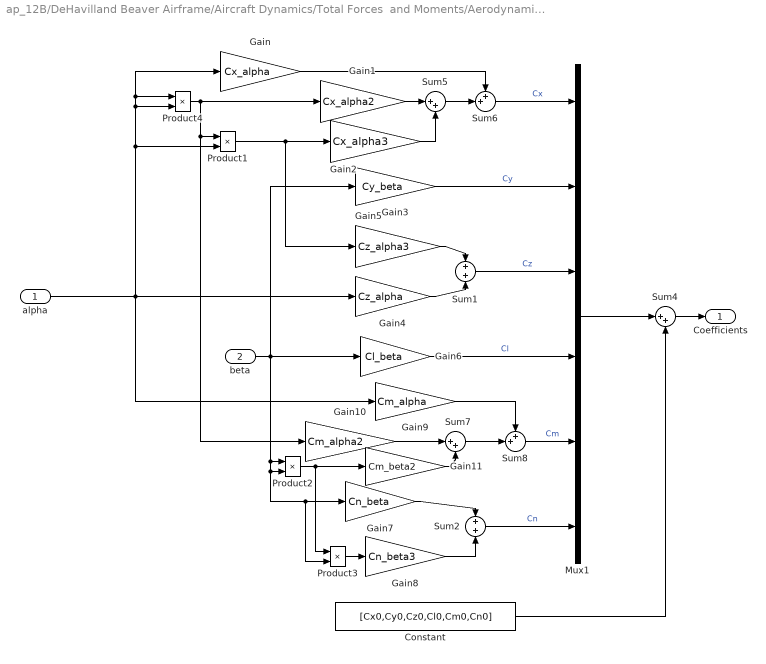
== system ap_12B/DeHavilland Beaver Airframe/Aircraft Dynamics/Total Forces  and Moments/Aerodynamics/Datum Coefficients ==
  alpha : Inport
  beta : Inport  Port=2
  Constant : Constant  Value=[Cx0,Cy0,Cz0,Cl0,Cm0,Cn0]
  Gain : Gain  Gain=Cx_alpha  SaturateOnIntegerOverflow=on  OutDataTypeStr=Inherit: Same as input  ParamDataTypeStr=Inherit: Same as input
  Gain1 : Gain  Gain=Cx_alpha2  SaturateOnIntegerOverflow=on  OutDataTypeStr=Inherit: Same as input  ParamDataTypeStr=Inherit: Same as input
  Gain10 : Gain  Gain=Cm_alpha2  SaturateOnIntegerOverflow=on  OutDataTypeStr=Inherit: Same as input  ParamDataTypeStr=Inherit: Same as input
  Gain11 : Gain  Gain=Cm_beta2  SaturateOnIntegerOverflow=on  OutDataTypeStr=Inherit: Same as input  ParamDataTypeStr=Inherit: Same as input
  Gain2 : Gain  Gain=Cx_alpha3  SaturateOnIntegerOverflow=on  OutDataTypeStr=Inherit: Same as input  ParamDataTypeStr=Inherit: Same as input
  Gain3 : Gain  Gain=Cy_beta  SaturateOnIntegerOverflow=on  OutDataTypeStr=Inherit: Same as input  ParamDataTypeStr=Inherit: Same as input
  Gain4 : Gain  Gain=Cz_alpha  SaturateOnIntegerOverflow=on  OutDataTypeStr=Inherit: Same as input  ParamDataTypeStr=Inherit: Same as input
  Gain5 : Gain  Gain=Cz_alpha3  SaturateOnIntegerOverflow=on  OutDataTypeStr=Inherit: Same as input  ParamDataTypeStr=Inherit: Same as input
  Gain6 : Gain  Gain=Cl_beta  SaturateOnIntegerOverflow=on  OutDataTypeStr=Inherit: Same as input  ParamDataTypeStr=Inherit: Same as input
  Gain7 : Gain  Gain=Cn_beta  SaturateOnIntegerOverflow=on  OutDataTypeStr=Inherit: Same as input  ParamDataTypeStr=Inherit: Same as input
  Gain8 : Gain  Gain=Cn_beta3  SaturateOnIntegerOverflow=on  OutDataTypeStr=Inherit: Same as input  ParamDataTypeStr=Inherit: Same as input
  Gain9 : Gain  Gain=Cm_alpha  SaturateOnIntegerOverflow=on  OutDataTypeStr=Inherit: Same as input  ParamDataTypeStr=Inherit: Same as input
  Mux1 : Mux  Inputs=6
  Product{1..4} (4 alike) : Product  SaturateOnIntegerOverflow=on  InputSameDT=on  OutDataTypeStr=Inherit: Same as first input
  Sum1 : Sum  SaturateOnIntegerOverflow=on
  Sum2 : Sum  SaturateOnIntegerOverflow=on
  Sum4 : Sum  Inputs=|++  SaturateOnIntegerOverflow=on
  Sum5 : Sum  Inputs=|++  SaturateOnIntegerOverflow=on
  Sum6 : Sum  Inputs=++|  SaturateOnIntegerOverflow=on
  Sum7 : Sum  Inputs=|++  SaturateOnIntegerOverflow=on
  Sum8 : Sum  Inputs=++|  SaturateOnIntegerOverflow=on
  Coefficients : Outport
  wires:
  Constant/1 -> Sum4/2
  Sum4/1 -> Coefficients/1
  Mux1/1 -> Sum4/1
  Gain10/1 -> Sum7/1
  Product2/1 -> Product3/1, Gain11/1
  Gain11/1 -> Sum7/2
  Gain9/1 -> Sum8/1
  Sum8/1 -> Mux1/5  "Cm"
  Product3/1 -> Gain8/1
  Gain8/1 -> Sum2/2
  Gain7/1 -> Sum2/1
  Gain5/1 -> Sum1/1
  Gain4/1 -> Sum1/2
  Product1/1 -> Gain5/1, Gain2/1
  Product4/1 -> Product1/1, Gain10/1, Gain1/1
  Gain/1 -> Sum6/1
  Sum2/1 -> Mux1/6  "Cn"
  Sum6/1 -> Mux1/1  "Cx"
  Sum1/1 -> Mux1/3  "Cz"
  Gain3/1 -> Mux1/2  "Cy"
  Gain6/1 -> Mux1/4  "Cl"
  alpha/1 -> Product1/2, Product4/2, Product4/1, Gain/1, Gain9/1, Gain4/1
  beta/1 -> Gain6/1, Gain3/1, Product3/2, Gain7/1, Product2/2, Product2/1
  Gain1/1 -> Sum5/1
  Gain2/1 -> Sum5/2
  Sum5/1 -> Sum6/2
  Sum7/1 -> Sum8/2

== system ap_12B/DeHavilland Beaver Airframe/Aircraft Dynamics/Total Forces  and Moments/Engine /eng ==
  note: dpt
  dpt : Inport
  alpha : Inport  Port=2
  Constant : Constant  Value=0
  Gain1 : Gain  Gain=Cn_dpt3  SaturateOnIntegerOverflow=on  OutDataTypeStr=Inherit: Same as input  ParamDataTypeStr=Inherit: Same as input
  Gain2 : Gain  Gain=Cm_dpt  SaturateOnIntegerOverflow=on  OutDataTypeStr=Inherit: Same as input  ParamDataTypeStr=Inherit: Same as input
  Gain3 : Gain  Gain=Cl_alpha2_dpt  SaturateOnIntegerOverflow=on  OutDataTypeStr=Inherit: Same as input  ParamDataTypeStr=Inherit: Same as input
  Gain4 : Gain  Gain=Cz_dpt  SaturateOnIntegerOverflow=on  OutDataTypeStr=Inherit: Same as input  ParamDataTypeStr=Inherit: Same as input
  Gain5 : Gain  Gain=Cx_dpt  SaturateOnIntegerOverflow=on  OutDataTypeStr=Inherit: Same as input  ParamDataTypeStr=Inherit: Same as input
  Gain6 : Gain  Gain=Cx_dpt2_alpha  SaturateOnIntegerOverflow=on  OutDataTypeStr=Inherit: Same as input  ParamDataTypeStr=Inherit: Same as input
  Mux2 : Mux  Inputs=6
  Product{,1..4,6} (6 alike) : Product  SaturateOnIntegerOverflow=on  OutDataTypeStr=Inherit: Same as first input
  Sum : Sum  Inputs=|++  SaturateOnIntegerOverflow=on
  Cprop : Outport
  wires:
  Sum/1 -> Mux2/1
  Gain6/1 -> Sum/2
  Gain5/1 -> Sum/1
  Constant/1 -> Mux2/2
  Gain4/1 -> Mux2/3
  Gain3/1 -> Mux2/4
  Gain2/1 -> Mux2/5
  Gain1/1 -> Mux2/6
  Product4/1 -> Gain3/1
  Product2/1 -> Gain6/1
  dpt/1 -> Gain5/1, Product/1, Product/2, Product6/2, Product1/2, Product1/1, Gain2/1, Gain4/1, Product4/2
  alpha/1 -> Product2/2, Product3/1, Product3/2
  Mux2/1 -> Cprop/1  "Cprop"
  Product/1 -> Product2/1
  Product3/1 -> Product4/1
  Product1/1 -> Product6/1
  Product6/1 -> Gain1/1

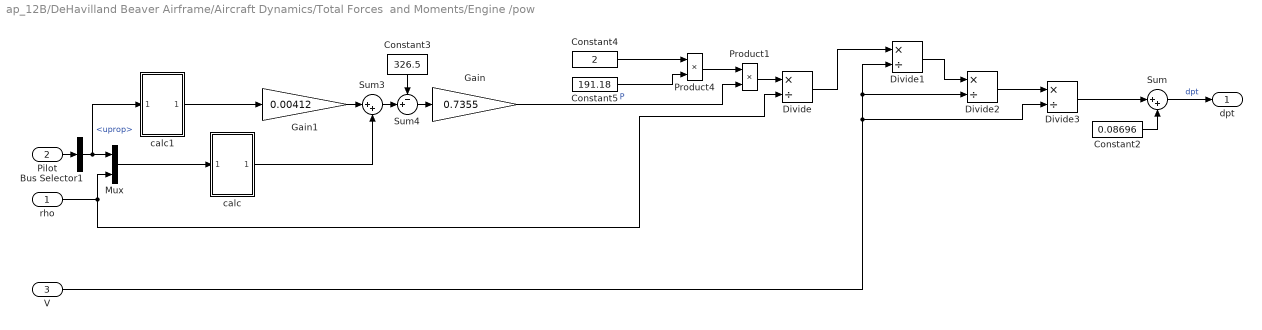
== system ap_12B/DeHavilland Beaver Airframe/Aircraft Dynamics/Total Forces  and Moments/Engine /pow ==
  rho : Inport
  Pilot : Inport  Port=2
  V : Inport  Port=3
  Bus Selector1 : BusSelector  OutputSignals=uprop
  Constant2 : Constant  Value=0.08696
  Constant3 : Constant  Value=326.5
  Constant4 : Constant  Value=2
  Constant5 : Constant  Value=191.18
  Divide{,1..3} (4 alike) : Product  Inputs=*/
  Gain : Gain  Gain=0.7355  SaturateOnIntegerOverflow=on  OutDataTypeStr=Inherit: Same as input  ParamDataTypeStr=Inherit: Same as input
  Gain1 : Gain  Gain=0.00412  SaturateOnIntegerOverflow=on  OutDataTypeStr=Inherit: Same as input  ParamDataTypeStr=Inherit: Same as input
  Mux : Mux  Inputs=2
  Product1 : Product  SaturateOnIntegerOverflow=on  OutDataTypeStr=Inherit: Same as first input
  Product4 : Product  SaturateOnIntegerOverflow=on  OutDataTypeStr=Inherit: Same as first input
  Sum : Sum  Inputs=|++  SaturateOnIntegerOverflow=on
  Sum3 : Sum  Inputs=|++  SaturateOnIntegerOverflow=on
  Sum4 : Sum  Inputs=-+|  SaturateOnIntegerOverflow=on
  calc : Subsystem
  calc1 : Subsystem
  dpt : Outport
  wires:
  calc/1(Out1) -> Sum3/2
  Constant3/1 -> Sum4/1
  Gain1/1 -> Sum3/1
  rho/1 -> Divide/2, Mux/2
  Sum/1 -> dpt/1  "dpt"
  V/1 -> Divide3/2, Divide1/2, Divide2/2
  Bus Selector1/1 -> calc1/1(In1), Mux/1  "<uprop>"
  Divide3/1 -> Sum/1
  Constant2/1 -> Sum/2
  Pilot/1 -> Bus Selector1/1
  Sum4/1 -> Gain/1
  Sum3/1 -> Sum4/2
  Mux/1 -> calc/1(In1)
  calc1/1(Out1) -> Gain1/1
  Constant4/1 -> Product4/1
  Constant5/1 -> Product4/2
  Product4/1 -> Product1/1
  Gain/1 -> Product1/2  "P"
  Product1/1 -> Divide/1
  Divide/1 -> Divide1/1
  Divide1/1 -> Divide2/1
  Divide2/1 -> Divide3/1

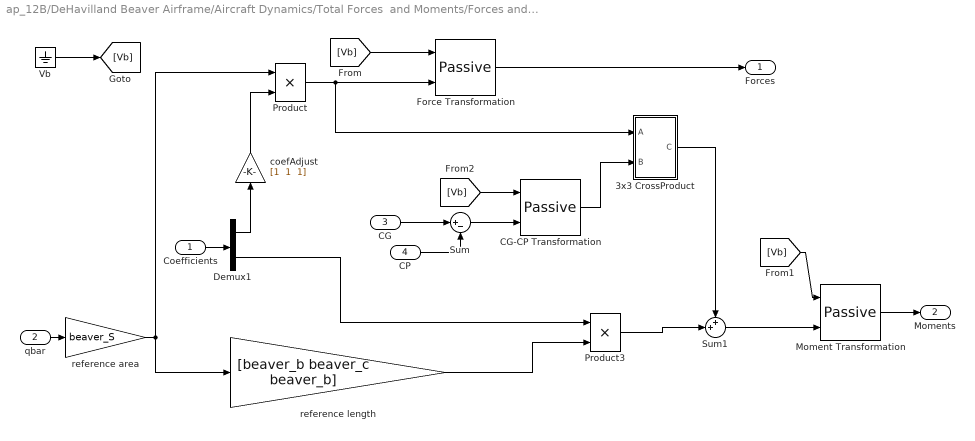
== system ap_12B/DeHavilland Beaver Airframe/Aircraft Dynamics/Total Forces  and Moments/Forces and Moments/Aero F&M ==
  Coefficients : Inport
  qbar : Inport  Port=2
  CG : Inport  Port=3
  CP : Inport  Port=4
  3x3 CrossProduct : Subsystem
  CG-CP Transformation : aerolibadynsys/Passive  SystemSampleTime=-1
  Demux1 : Demux  Outputs=[3,3]
  Force Transformation : aerolibadynsys/Passive  SystemSampleTime=-1
  Moment Transformation : aerolibadynsys/Passive  SystemSampleTime=-1
  Product : Product  SaturateOnIntegerOverflow=on  InputSameDT=on  OutDataTypeStr=Inherit: Same as first input
  Product3 : Product  SaturateOnIntegerOverflow=on  InputSameDT=on  OutDataTypeStr=Inherit: Same as first input
  Sum : Sum  Inputs=|+-  SaturateOnIntegerOverflow=on
  Sum1 : Sum  Inputs=++|  SaturateOnIntegerOverflow=on  InputSameDT=on  OutDataTypeStr=Inherit: Same as first input
  Vb : Ground
  coefAdjust : Gain  Gain="[1  1  1]"
  reference area : Gain  Gain=beaver_S  SaturateOnIntegerOverflow=on  OutDataTypeStr=Inherit: Same as input  ParamDataTypeStr=Inherit: Same as input
  reference length : Gain  Gain=[beaver_b beaver_c beaver_b]  SaturateOnIntegerOverflow=on  OutDataTypeStr=Inherit: Same as input  ParamDataTypeStr=Inherit: Same as input
  Forces : Outport
  Moments : Outport  Port=2
  wires:
  [Vb] -> Force Transformation/1
  CP/1 -> Sum/2
  reference length/1 -> Product3/2
  Demux1/2 -> Product3/1
  qbar/1 -> reference area/1
  coefAdjust/1 -> Product/2
  Force Transformation/1 -> Forces/1
  Demux1/1 -> coefAdjust/1
  Coefficients/1 -> Demux1/1
  [Vb] -> Moment Transformation/1
  [Vb] -> CG-CP Transformation/1
  CG-CP Transformation/1 -> 3x3 CrossProduct/2(B)
  Product3/1 -> Sum1/2
  Vb/1 -> [Vb]
  reference area/1 -> reference length/1, Product/1
  Moment Transformation/1 -> Moments/1
  Product/1 -> 3x3 CrossProduct/1(A), Force Transformation/2
  Sum/1 -> CG-CP Transformation/2
  Sum1/1 -> Moment Transformation/2
  3x3 CrossProduct/1(C) -> Sum1/1
  CG/1 -> Sum/1

== system ap_12B/DeHavilland Beaver Airframe/Aircraft Dynamics/6DoF (Quaternion)/Calculate DCM & Euler Angles/Quaternions to  Direction Cosine Matrix/Quaternion Normalize ==
  q : Inport
  Demux : Demux
  Mux : Mux
  Product{,1..3} (4 alike) : Product  Inputs=*/
  Quaternion Modulus : Subsystem
  normal(q) : Outport
  wires:
  Product3/1 -> Mux/4
  Product1/1 -> Mux/2
  Demux/1 -> Product/1
  Quaternion Modulus/1(|q|) -> Product1/2, Product/2, Product2/2, Product3/2
  Mux/1 -> normal(q)/1
  q/1 -> Quaternion Modulus/1(q), Demux/1
  Product/1 -> Mux/1
  Demux/3 -> Product2/1
  Demux/4 -> Product3/1
  Product2/1 -> Mux/3
  Demux/2 -> Product1/1

== system ap_12B/DeHavilland Beaver Airframe/Aircraft Dynamics/6DoF (Quaternion)/Calculate DCM & Euler Angles/Quaternions to Rotation Angles (ZYX)/Quaternion Normalize ==
  q : Inport
  Demux : Demux
  Mux : Mux
  Product{,1..3} (4 alike) : Product  Inputs=*/
  Quaternion Modulus : Subsystem
  normal(q) : Outport
  wires:
  Product3/1 -> Mux/4
  Product1/1 -> Mux/2
  Demux/1 -> Product/1
  Quaternion Modulus/1(|q|) -> Product1/2, Product/2, Product2/2, Product3/2
  Mux/1 -> normal(q)/1
  q/1 -> Quaternion Modulus/1(q), Demux/1
  Product/1 -> Mux/1
  Demux/3 -> Product2/1
  Demux/4 -> Product3/1
  Product2/1 -> Mux/3
  Demux/2 -> Product1/1

== system ap_12B/DeHavilland Beaver Airframe/Aircraft Dynamics/Total Forces  and Moments/Actuators/sof/ResetIntegratorInternal ==
  note: ic
  note: Level Reset Integration With Saturation
      | y(n) = y(n-1) + K*Ts*u(n-1)
  U : Inport
  R : Inport  Port=2
  ic : Inport  Port=3
  Constant : Constant  Value=1.0
  Constant1 : Constant  Value=Ts
  Product : Product  RndMeth=Zero
  Product1 : Product  RndMeth=Zero
  Sum3 : Sum
  Switch : Switch  Criteria=u2 ~= 0
  Switch1 : Switch  Criteria=u2 ~= 0
  X : UnitDelay  SampleTime=Ts
  Y : Outport
  wires:
  Product1/1 -> Sum3/1
  U/1 -> Product1/2
  Sum3/1 -> Switch1/3
  Product/1 -> Product1/1
  ic/1 -> Switch1/1, Switch/1
  Constant1/1 -> Product/2  "deltaT"
  Switch1/1 -> X/1
  Constant/1 -> Product/1  "gain"
  Switch/1 -> Y/1, Sum3/2
  R/1 -> Switch1/2, Switch/2
  X/1 -> Switch/3
